simulink model "Task8"  (R2025a)
settings: Solver=VariableStepAuto  StartTime=0.0  StopTime=10.0  RelTol=1e-3
settings Model: Creator=LOQ  LastModifiedBy=LOQ

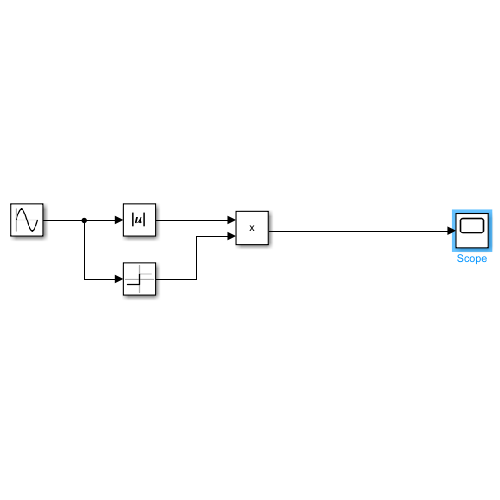
[thumbnail: Simulink's stored preview of the top-level diagram]
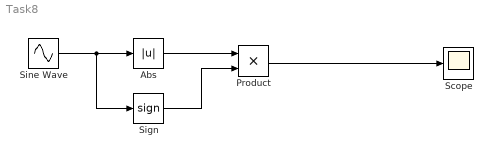
== system Task8 ==
  Abs : Abs  SaturateOnIntegerOverflow=off
  Product : Product
  Scope : Scope
      settings: ActiveDisplayYMinimum=-1.2494670038018805  ActiveDisplayYMaximum=1.2494670038018814
  Sign : Signum
  Sine Wave : Sin  SampleTime=0
  wires:
  Sine Wave/1 -> Sign/1, Abs/1
  Abs/1 -> Product/1
  Sign/1 -> Product/2
  Product/1 -> Scope/1
